simulink model "forceControlInnerVelocity"  (R2021a)
settings: Solver=VariableStepAuto  StartTime=0.0  StopTime=25  RelTol=1e-3
values from neighbouring files (symbols this model uses):
  C_f_P_vel = K_f_vel    [assignment14_main.m]
  f_d = [0 -0.5 0.1].'    [assignment14_main.m]
  K = diag([0 10 0])    [assignment14_main.m]
  K_f_vel = 0.1*diag([10 10 10])    [assignment14_main.m]
  K_i_vel = 0.05*diag([10 10 10])    [assignment14_main.m]
  Kd_vel = 4*diag([10, 10, 10])    [assignment14_main.m]
  Kp_vel = 3*diag([10, 10, 10])    [assignment14_main.m]
  M_d = 0.1*diag([10 10 10])    [assignment14_main.m]
libraries: vrlib x1
settings Model: Creator=fabio  LastModifiedBy=fabio

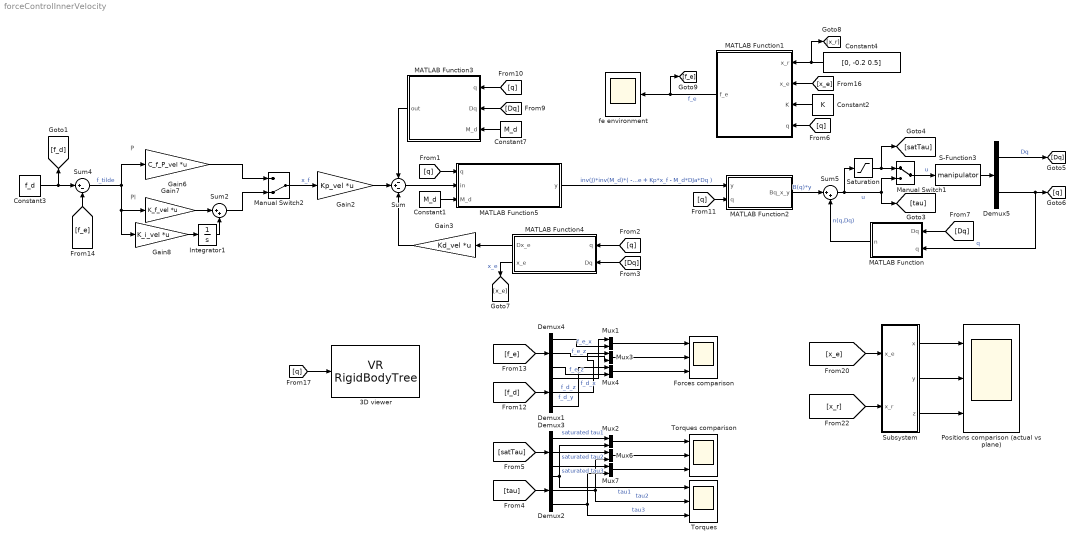
== system forceControlInnerVelocity ==
  note: PI
  note: P
  3D viewer : vrlib/VR RigidBodyTree  RBT=robot  useRBT=off  Ts=0.5  ForceViewerOpen=on
      settings: SourceProductBaseCode=SL
  Constant1 : Constant  Value=M_d  VectorParams1D=off
  Constant2 : Constant  Value=K  VectorParams1D=off
  Constant3 : Constant  Value=f_d
  Constant4 : Constant  Value=[0, -0.2 0.5]
  Constant7 : Constant  Value=M_d  VectorParams1D=off
  Demux{1..4} (4 alike) : Demux  Outputs=3
  Demux5 : Demux  Outputs=[3 3]
  Forces comparison : Scope  NumInputPorts=3
  Gain2 : Gain  Gain=Kp_vel  Multiplication=Matrix(K*u) (u vector)
  Gain3 : Gain  Gain=Kd_vel  Multiplication=Matrix(K*u) (u vector)
  Gain6 : Gain  Gain=C_f_P_vel  Multiplication=Matrix(K*u)
  Gain7 : Gain  Gain=K_f_vel  Multiplication=Matrix(K*u)
  Gain8 : Gain  Gain=K_i_vel  Multiplication=Matrix(K*u)
  Integrator1 : Integrator
  MATLAB Function : MATLAB Function  TreatAsAtomicUnit=on
  MATLAB Function1 : MATLAB Function  TreatAsAtomicUnit=on
  MATLAB Function2 : MATLAB Function  TreatAsAtomicUnit=on
  MATLAB Function3 : MATLAB Function  TreatAsAtomicUnit=on
  MATLAB Function4 : MATLAB Function  TreatAsAtomicUnit=on
  MATLAB Function5 : MATLAB Function  TreatAsAtomicUnit=on
  Manual Switch1 : ManualSwitch
  Manual Switch2 : ManualSwitch  CurrentSetting=0
  Mux{1..4,6..7} (6 alike) : Mux  Inputs=2
  Positions comparison (actual vs plane) : Scope  NumInputPorts=3
  S-Function3 : S-Function  FunctionName=manipulator  Parameters=myRobot  SFunctionDeploymentMode=off  EnableBusSupport=off
  Saturation : Saturate  UpperLimit=20  LowerLimit=-20
  Subsystem : Subsystem
  Sum : Sum  Inputs=-+-
  Sum2 : Sum  Inputs=|++
  Sum4 : Sum  Inputs=|+-
  Sum5 : Sum  Inputs=|++
  Torques : Scope  NumInputPorts=3
  Torques comparison : Scope  NumInputPorts=3
  fe environment : Scope
  wires:
  Manual Switch1/1 -> S-Function3/1  "u"
  S-Function3/1 -> Demux5/1
  Demux5/1 -> [Dq]  "Dq"
  Demux5/2 -> MATLAB Function/2(q), [q]  "q"
  Gain2/1 -> Sum/2
  Sum/1 -> MATLAB Function5/2(in)
  MATLAB Function2/1(Bq_x_y) -> Sum5/1  "B(q)*y"
  Demux2/1 -> Torques/1, Mux2/2  "tau1"
  [tau] -> Demux2/1
  Saturation/1 -> [satTau], Manual Switch1/1
  [satTau] -> Demux3/1
  Demux3/1 -> Mux2/1  "saturated tau1"
  Mux2/1 -> Torques comparison/1
  Mux6/1 -> Torques comparison/2
  Mux7/1 -> Torques comparison/3
  Demux2/2 -> Torques/2, Mux6/2  "tau2"
  Demux3/2 -> Mux6/1  "saturated tau2"
  Demux3/3 -> Mux7/1  "saturated tau3"
  Demux2/3 -> Torques/3, Mux7/2  "tau3"
  Sum5/1 -> Manual Switch1/2, [tau], Saturation/1  "u"
  MATLAB Function4/2(x_e) -> [x_e]  "x_e"
  [Dq] -> MATLAB Function/1(Dq)
  [Dq] -> MATLAB Function3/2(Dq)
  [q] -> MATLAB Function3/1(q)
  [q] -> MATLAB Function2/2(q)
  [q] -> 3D viewer/1
  [q] -> MATLAB Function5/1(q)
  MATLAB Function5/1(y) -> MATLAB Function2/1(y)  "inv(J)*inv(M_d)*( -Kd*Dx_e + Kp*x_f - M_d*DJa*Dq )"
  [q] -> MATLAB Function4/1(q)
  [Dq] -> MATLAB Function4/2(Dq)
  MATLAB Function4/1(Dx_e) -> Gain3/1
  Gain3/1 -> Sum/3
  Constant7/1 -> MATLAB Function3/3(M_d)
  MATLAB Function3/1(out) -> Sum/1
  Constant4/1 -> [x_r], MATLAB Function1/1(x_r)
  [x_e] -> MATLAB Function1/2(x_e)
  Constant2/1 -> MATLAB Function1/3(K)
  MATLAB Function/1(n) -> Sum5/2  "n(q,Dq)"
  MATLAB Function1/1(f_e) -> fe environment/1, [f_e]  "f_e"
  Constant3/1 -> [f_d], Sum4/1
  [q] -> MATLAB Function1/4(q)
  Demux1/3 -> Mux4/1  "f_d_z"
  Demux4/3 -> Mux4/2  "f_e_z"
  Demux4/2 -> Mux3/2  "f_e_z"
  Demux1/2 -> Mux3/1  "f_d_y"
  Mux4/1 -> Forces comparison/3
  Mux3/1 -> Forces comparison/2
  Mux1/1 -> Forces comparison/1
  Demux4/1 -> Mux1/2  "f_e_x"
  [f_e] -> Demux4/1
  [f_d] -> Demux1/1
  Demux1/1 -> Mux1/1  "f_d_x"
  Constant1/1 -> MATLAB Function5/3(M_d)
  Subsystem/2(y) -> Positions comparison (actual vs plane)/2
  Subsystem/1(x) -> Positions comparison (actual vs plane)/1
  Subsystem/3(z) -> Positions comparison (actual vs plane)/3
  [x_r] -> Subsystem/2(x_r)
  [x_e] -> Subsystem/1(x_e)
  [f_e] -> Sum4/2
  Manual Switch2/1 -> Gain2/1  "x_f"
  Gain8/1 -> Integrator1/1
  Sum2/1 -> Manual Switch2/2
  Gain6/1 -> Manual Switch2/1
  Integrator1/1 -> Sum2/2
  Gain7/1 -> Sum2/1
  Sum4/1 -> Gain6/1, Gain8/1, Gain7/1  "f_tilde"

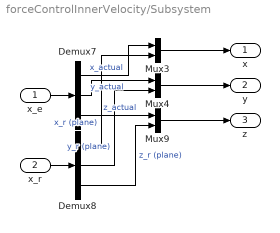
== system forceControlInnerVelocity/Subsystem ==
  x_e : Inport
  x_r : Inport  Port=2
  Demux7 : Demux  Outputs=3
  Demux8 : Demux  Outputs=3
  Mux3 : Mux  Inputs=2
  Mux4 : Mux  Inputs=2
  Mux9 : Mux  Inputs=2
  x : Outport
  y : Outport  Port=2
  z : Outport  Port=3
  wires:
  Demux8/1 -> Mux3/2  "x_r (plane)"
  Demux7/3 -> Mux9/1  "z_actual"
  Demux8/2 -> Mux4/2  "y_r (plane)"
  Demux7/1 -> Mux3/1  "x_actual"
  Demux8/3 -> Mux9/2  "z_r (plane)"
  Demux7/2 -> Mux4/1  "y_actual"
  x_e/1 -> Demux7/1
  Mux9/1 -> z/1
  Mux4/1 -> y/1
  Mux3/1 -> x/1
  x_r/1 -> Demux8/1

== matlab function forceControlInnerVelocity/MATLAB Function1 ==
  data: x_r input; x_e input; K input; f_e output; q input
function f_e = environment(x_r, x_e, K, q)    
    
    y_plane = x_r(2);
    
    %contact with the plane
    if max(size(x_e)) > 1 && x_e(2) < y_plane 
        f_e = K*(x_e - x_r);
        
    else %no contact with the plane
        f_e = [0 0 0].';
    end   
end

== matlab function forceControlInnerVelocity/MATLAB Function ==
  data: Dq input; n output; q input
function n = n_q_Dq(Dq, q)
    
    %To get the "perfect" matrices use the following code
    C = get_C_matrix(q,Dq);
    G = get_G_matrix(q);
    
    
    %To get the "wrongly estimated" matrices use the following code   
%     theta2 = q(2);   d3 = q(3); 
%     Dtheta2 = Dq(2); Dd3 = Dq(3); 
%     
%     m_Link4 = 0.16;  %0.2kg is the correct value
% 
%     C = [0,                         0,                        0;
%          0,            m_Link4*Dd3*d3,       m_Link4*Dtheta2*d3;
%          0,       -m_Link4*Dtheta2*d3,                        0];
%    
%     G = [           0                           ;
%          (981*m_Link4*sin(theta2)*d3)/100 ;
%           -(981*m_Link4*cos(theta2))/100    ];


    
    n = C*Dq + G; %F = friction is neglected

end

== matlab function forceControlInnerVelocity/MATLAB Function2 ==
  data: y input; Bq_x_y output; q input
function Bq_x_y = Bq_x_y(y,q)
    Bq_x_y = get_B_matrix(q)*y;
end

== matlab function forceControlInnerVelocity/MATLAB Function3 ==
  data: q input; out output; Dq input; M_d input
function out = M_d_x_DJa_x_Dq(q, Dq, M_d)
    if max(size(q)) < 3
        q = [0 0 0];   
    end
    if max(size(Dq)) < 3
        Dq = [0 0 0];   
    end
    
    %Get DJa from ∑0 to ∑ee 
    DJa = get_DJa_matrix(q, Dq);
    DJa = DJa(1:3,1:3); %only the linear components are considered!     

    out = M_d * DJa * Dq;
      
end

== matlab function forceControlInnerVelocity/MATLAB Function4 ==
  data: Dx_e output; q input; x_e output; Dq input
function [Dx_e, x_e] = k(q, Dq) 
    %Compute the direct kinematics from last transformation matrix
    if max(size(q)) < 3
        q = [0 0 0];   
    end
    if max(size(Dq)) < 3
        Dq = [0 0 0];   
    end
    
    %get translation vector from ∑0 to ∑ee   
    T0_to_ee = get_T0_ee_matrix(q);
    p0_to_ee = T0_to_ee(1:3,4);        
  
    x_e = [ p0_to_ee ]; %orientation isn't considered!
      
    Ja = get_Ja_matrix(q);
    Ja = Ja(1:3,1:3); %only the linear components are considered!
    Dx_e = Ja * Dq;
end

== matlab function forceControlInnerVelocity/MATLAB Function5 ==
  data: q input; y output; in input; M_d input
function y = invJa_x_invMd_x_in(q, in, M_d)
    if max(size(q)) < 3
        q = [0 0 0];   
    end
    
    Ja = get_Ja_matrix(q);
    Ja = Ja(1:3,1:3); %only the linear components are considered!     
    
    y = pinv(Ja) * pinv(M_d) * in;
 
end
